simulink model "ANC_simulink_3"  (R2023b)
settings: Solver=VariableStepAuto  StartTime=0.0  StopTime=10.0  RelTol=1e-3
values from neighbouring files (symbols this model uses):
  A = 10    [parameter.mat]
  c = 343    [parameter.mat]
  f = 10    [parameter.mat]
  Lp = 1    [parameter.mat]
  Ls = 0.1    [parameter.mat]
  Ts = 0.001    [parameter.mat]
settings Model: Creator=nurbi  LastModifiedBy=nurbi

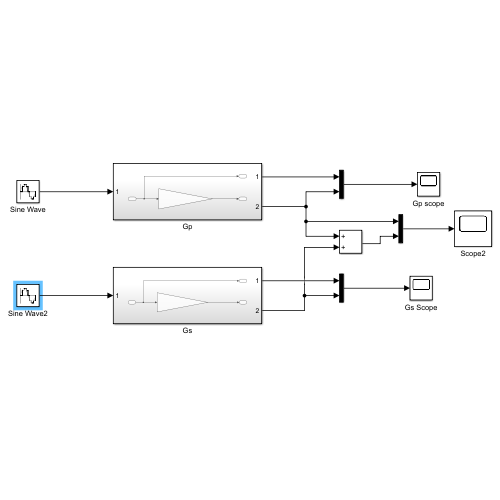
[thumbnail: Simulink's stored preview of the top-level diagram]
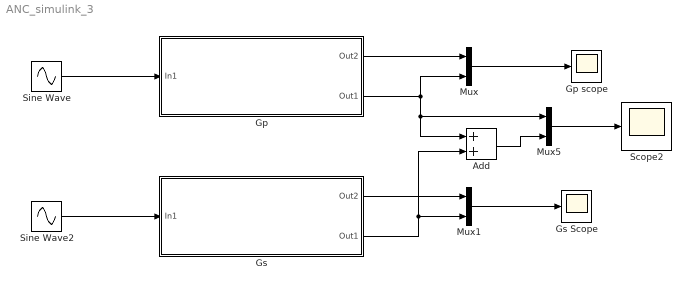
== system ANC_simulink_3 ==
  Add : Sum
  Gp : Subsystem
  Gp scope : Scope
  Gs : Subsystem
  Gs Scope : Scope
  Mux : Mux  Inputs=2
  Mux1 : Mux  Inputs=2
  Mux5 : Mux  Inputs=2
  Scope2 : Scope
  Sine Wave : Sin  Amplitude=A  Frequency=2*pi*f  SampleTime=Ts
  Sine Wave2 : Sin  Amplitude=5  Frequency=2*pi*f  SampleTime=Ts
  wires:
  Sine Wave2/1 -> Gs/1(In1)
  Sine Wave/1 -> Gp/1(In1)
  Mux/1 -> Gp scope/1
  Add/1 -> Mux5/2
  Mux5/1 -> Scope2/1
  Mux1/1 -> Gs Scope/1
  Gs/2(Out1) -> Mux1/2, Add/2
  Gp/2(Out1) -> Add/1, Mux5/1, Mux/2
  Gp/1(Out2) -> Mux/1
  Gs/1(Out2) -> Mux1/1

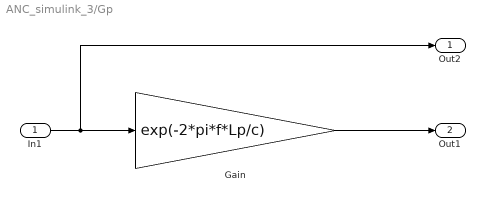
== system ANC_simulink_3/Gp ==
  In1 : Inport
  Gain : Gain  Gain=exp(-2*pi*f*Lp/c)
  Out2 : Outport
  Out1 : Outport  Port=2
  wires:
  In1/1 -> Out2/1, Gain/1
  Gain/1 -> Out1/1

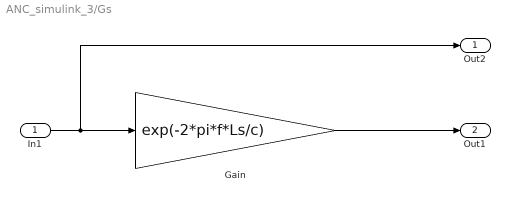
== system ANC_simulink_3/Gs ==
  In1 : Inport
  Gain : Gain  Gain=exp(-2*pi*f*Ls/c)
  Out2 : Outport
  Out1 : Outport  Port=2
  wires:
  In1/1 -> Out2/1, Gain/1
  Gain/1 -> Out1/1
